simulink model "pwm"  (R2023a)
settings: Solver=VariableStepAuto  StartTime=0.0  StopTime=20  RelTol=1e-3
undefined symbols (not defined in the file): Acid, Lead
libraries: spsSeriesRLCBranchLib x3, spsBatteryLib x1, spsCurrentMeasurementLib x1, spsDiodeLib x1, spsMosfetLib x1, spsPVArrayLib x1, eePwmGenerator x1, simulink x1, spsVoltageMeasurementLib x1, spspowerguiLib x1
settings Model: SimulationMode=rapid-accelerator  Creator=mluser  LastModifiedBy=mluser
settings SolverCC: ZeroCrossAlgorithm=Adaptive
settings DebuggingCC: IgnoredZcDiagnostic=none

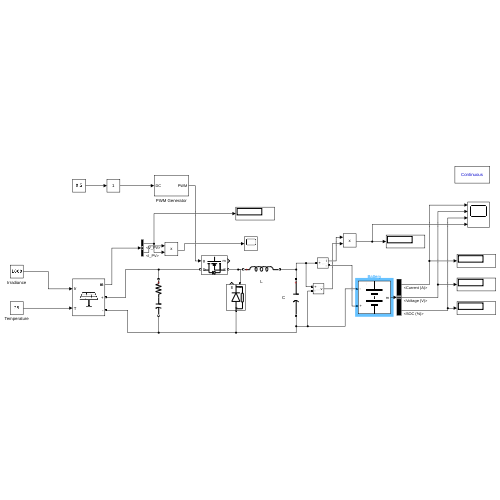
[thumbnail: Simulink's stored preview of the top-level diagram]
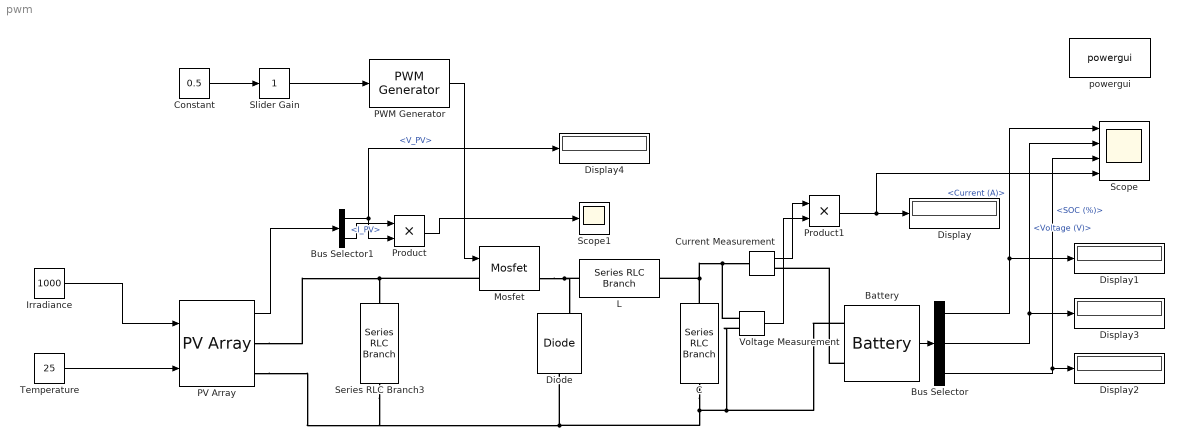
== system pwm ==
  Battery : spsBatteryLib/Battery  BatType=Lead-Acid  ShowTempParam=off  ThermalPreset=no  ShowAgeParam=off  NomV=12  NomQ=10  SOC=99.6  Batt_Tr=30  PresetModel=on  MaxQ=10.4167  MinV=9  FullV=13.0658  Dis_rate=2  R=0.012  Normal_OP=3.1028  expZone="[12.2171    0.0333333]"  current=[6.5 13 32.5]  Units=Time  Tci=20  NomT=20  T2=-30  MaxQ2=4.8  FullV2=7.1  Normal_OP2=5.655  expZone2="[6.58           1]"  Rca=0.6  ti=2000  Dp=0  Neq0=0  Tsim=1e6  Ta1=25  Qeol=5.4*0.9  Reol=0.013333*1.2  Char_age=[2.3478, 3]  Dis_age=[2.3478, 10]  N1=1500  N2=10500  N3=1000  N4=1400  Ta2=45  N5=950
  Bus Selector : BusSelector  OutputSignals=Current (A),Voltage (V),SOC (%)
  Bus Selector1 : BusSelector  OutputSignals=V_PV,I_PV
  C : spsSeriesRLCBranchLib/Series RLC Branch  LConnTagsString=__new0  RConnTagsString=__new0  BranchType=C  Resistance=1  Inductance=1e-3  SetiL0=off  InitialCurrent=0  Capacitance=1000e-6  Setx0=off  InitialVoltage=0  Measurements=None
  Constant : Constant  Value=0.5
  Current Measurement : spsCurrentMeasurementLib/Current Measurement  PhasorSimulation=off  OutputType=Complex  PSBequivalent=0
  Diode : spsDiodeLib/Diode  Ron=0.001  Lon=0  Vf=0.8  IC=0  UseSnubber=0  Rs=500  Cs=250e-9  Measurements=on
  Display{,1..4} (5 alike) : Display
  Irradiance : Constant  Value=1000
  L : spsSeriesRLCBranchLib/Series RLC Branch  LConnTagsString=__new0  RConnTagsString=__new0  BranchType=L  Resistance=1  Inductance=100e-6  SetiL0=off  InitialCurrent=0  Capacitance=1e-6  Setx0=off  InitialVoltage=0  Measurements=None
  Mosfet : spsMosfetLib/Mosfet  Ron=0.1  Lon=0  Rd=0.01  Vfd=0  IC=0  Rs=1e5  Cs=inf  Measurements=on
  PV Array : spsPVArrayLib/PV Array  Npar=1  Nser=1  PlotType=array @ 1000 W/m2 & specified temperatures  S_vec="[ 1000  500  100 ]"  Temp_C_vec="[ 45 25  ]"  ModuleName=Canadian Solar Inc. CS5A-180MX  PlotWhenSelected=off  Pm=180.139  Ncell=72  Voc=44.5  Isc=5.4  Vm=36.1  Im=4.99  beta_Voc_pc=-0.374  alpha_Isc_pc=0.089  beta_Voc=-0.16643  alpha_Isc=0.004806  IL=5.4115  I0=3.053e-10  nI=1.0208  Rsh=268.1861  Rs=0.56943  RobustModel=off  RobustCellTemperature=313.3991  BAL=on  Tc=1e-6  Tfilter=5e-5
  PWM Generator : eePwmGenerator/PWM Generator  CarrCount=Up  Tper=0.001  Tdelay=0  Ts=0.25e-6
  Product : Product
  Product1 : Product
  Scope : Scope  NumInputPorts=4
  Scope1 : Scope
  Series RLC Branch3 : spsSeriesRLCBranchLib/Series RLC Branch  LConnTagsString=__new0  RConnTagsString=__new0  BranchType=RC  Resistance=0.001  Inductance=1e-3  SetiL0=off  InitialCurrent=0  Capacitance=0.001  Setx0=off  InitialVoltage=0  Measurements=None
  Slider Gain : simulink/Math Operations/Slider Gain  gain=1  low=0  high=2
  Temperature : Constant  Value=25
  Voltage Measurement : spsVoltageMeasurementLib/Voltage Measurement  PhasorSimulation=off  OutputType=Complex  PSBequivalent=0
  powergui : spspowerguiLib/powergui  Priority=1  SimulationMode=Continuous  SampleTime=1e-6  frequency=60  Iterations=50  frequencyindice=0  Pbase=100e6  ErrMax=1e-4  UnitsV=kV  UnitsW=MW  buscounter=0  FunctionMessages=off  echomessages=off  EnableUseOfTLC=off  CurrentSourceSwitches=off  DisableSnubberDevices=off  DisableRonSwitches=off  DisableVfSwitches=off  DisplayEquations=off  AutomaticDiscreteSolvers=off  SolverType=Tustin/Backward Euler (TBE)  Interpol=off  ExternalGateDelay=off  methode=off  Ts=100  x0status=blocks  SPID=on  SwTol=0  HookPort=off  NonlinearTolerance=1e-4  nMaxIteration=100  ContinueOnMaxIteration=off  RestoreLinks=warning  ResistiveCurrentMeasurement=off  Frange=[0:2:500]  Ylog=off  Xlog=on  ShowGrid=off  save=off  variable=ZData  structure=0  ZoomFFT=off  StartTime=0.0  cycles=1  DisplayStyle=1  fundamental=60  FreqAxis=off  MaxFrequency=1000  frequencyindicesteady=1  RmsSteady=1  display=off
  wires:
  Battery/1 -> Bus Selector/1
  Bus Selector/2 -> Scope/2, Display3/1  "<Voltage (V)>"
  Bus Selector/3 -> Scope/3, Display2/1  "<SOC (%)>"
  Temperature/1 -> PV Array/2
  Irradiance/1 -> PV Array/1
  Bus Selector/1 -> Scope/1, Display1/1  "<Current (A)>"
  PV Array/1 -> Bus Selector1/1
  Bus Selector1/1 -> Display4/1, Product/2  "<V_PV>"
  Bus Selector1/2 -> Product/1  "<I_PV>"
  PWM Generator/1 -> Mosfet/1
  Product/1 -> Scope1/1
  Constant/1 -> Slider Gain/1
  Slider Gain/1 -> PWM Generator/1
  Current Measurement/1 -> Product1/1
  Voltage Measurement/1 -> Product1/2
  Product1/1 -> Scope/4, Display/1
  connections:
  Mosfet/RConn1 -- Diode/RConn1 -- L/LConn1
  Battery/LConn2 -- Voltage Measurement/LConn2 -- C/RConn1 -- Series RLC Branch3/RConn1 -- PV Array/RConn2 -- Diode/LConn1
  C/LConn1 -- Voltage Measurement/LConn1 -- Current Measurement/LConn1 -- L/RConn1
  Mosfet/LConn1 -- Series RLC Branch3/LConn1 -- PV Array/RConn1
  Battery/LConn1 -- Current Measurement/RConn1
